simulink library "monroe_library"  (R2012b)
settings: Solver=ode45  StartTime=0.0  StopTime=10.0  RelTol=1e-3
values from neighbouring files (symbols this model uses):
  input_bit_width = ', num2str(input_bit_width))    [fft_direct_draw.m]
undefined symbols (not defined in the file or in its folder): gcbh, xlBlockLoadCallback
libraries: xbsIndex_r4 x1880, monroe_library x159, casper_library x13, xps_library x1
(part 22 of 43)

== system monroe_library/direct_coeff_gen/coeff_gen_stage_3_group_1 ==
  sync : Inport
  Concat : xbsIndex_r4/Concat  num_inputs=2  dbl_ovrd=off  block_type=concat
  Concat1 : xbsIndex_r4/Concat  num_inputs=2  dbl_ovrd=off  block_type=concat
  Concat2 : xbsIndex_r4/Concat  num_inputs=2  dbl_ovrd=off  block_type=concat
  Constant : xbsIndex_r4/Constant  arith_type=Boolean  const=0  n_bits=16  bin_pt=14  explicit_period=on  period=1  equ=P=C  opselect=C  inp2=PCIN>>17  opr=+  inp1=P  carry=CIN  dbl_ovrd=off  block_type=constant
  Constant1 : xbsIndex_r4/Constant  arith_type=Boolean  const=1  n_bits=16  bin_pt=14  explicit_period=off  period=1  equ=P=C  opselect=C  inp2=PCIN>>17  opr=+  inp1=P  carry=CIN  dbl_ovrd=off  block_type=constant
  Constant3 : xbsIndex_r4/Constant  arith_type=Signed (2's comp)  const=0  n_bits=18  bin_pt=17  explicit_period=on  period=1  equ=P=C  opselect=C  inp2=PCIN>>17  opr=+  inp1=P  carry=CIN  dbl_ovrd=off  block_type=constant
  Constant4 : xbsIndex_r4/Constant  arith_type=Boolean  const=0  n_bits=16  bin_pt=14  explicit_period=off  period=1  equ=P=C  opselect=C  inp2=PCIN>>17  opr=+  inp1=P  carry=CIN  dbl_ovrd=off  block_type=constant
  Constant5 : xbsIndex_r4/Constant  arith_type=Unsigned  const=2  n_bits=10  bin_pt=0  explicit_period=on  period=1  equ=P=C  opselect=C  inp2=PCIN>>17  opr=+  inp1=P  carry=CIN  dbl_ovrd=off  block_type=constant
  Counter : xbsIndex_r4/Counter  cnt_type=Free Running  cnt_to=Inf  operation=Up  start_count=0  cnt_by_val=1  arith_type=Unsigned  n_bits=10  bin_pt=0  load_pin=on  rst=off  en=off  explicit_period=on  period=1  dbl_ovrd=off  use_behavioral_HDL=off  implementation=Fabric  block_type=counter
  Delay : xbsIndex_r4/Delay  en=off  latency=0  dbl_ovrd=off  reg_retiming=off  block_type=delay
  Dual Port RAM4 : xbsIndex_r4/Dual Port RAM  depth=2048  initVector=[0 -0.000766990318742704 -0.00153398018628477 -0.0023009691514258 -0.00306795676296598 -0.00383494256970623 -0.00460192612044857 -0.00536890696399634 -0.00613588464915448 -0.00690285872472976 -0.0076698287395311 -0.0084367942423698 -0.00920375478205982 -0.00997070990741803 -0.0107376591672645 -0.0115046021104227 -0.0122715382857199 -0.0130384672419873 -0.0138053885280604 -0.0145723016927791 -0.0153392062849881 -0.0161061018535373 -0.0168729879472817 -0.0176398641150821 -0.0184067299058048 -0.0191735848683226 -0.0199404285515144 -0.0207072605042659 -0.0214740802754695 -0.022240887414025 -0.0230076814688394 -0.0237744619888276 -0.0245412285229123 -0.0253079806200246 -0.0260747178291039 -0.0268414396990985 -0.0276081457789657 -0.0283748356176721 -0.0291415087641937 -0.0299081647675166 -0.0306748031766366 -0.0314414235405603 -0.0322080254083046 -0.0329746083288973 -0.0337411718513776 -0.0345077155247957 -0.0352742388982139 -0.0360407415207062 -0.0368072229413588 -0.0375736827092705 -0.0383401203735527 -0.0391065354833299 -0.0398729275877398 -0.0406392962359337 -0.0414056409770767 -0.0421719613603479 -0.0429382569349408 -0.0437045272500634 -0.0444707718549387 -0.0452369902988046 -0.0460031821309146 -0.0467693469005379 -0.0475354841569593 -0.0483015934494801 -0.049067674327418 -0.0498337263401073 -0.0505997490368993 -0.0513657419671626 -0.0521317046802833 -0.0528976367256653 -0.0536635376527305 -0.0544294070109191 -0.0551952443496899 -0.0559610492185206 -0.0567268211669077 -0.0574925597443676 -0.0582582645004358 -0.0590239349846679 -0.0597895707466399 -0.0605551713359478 -0.0613207363022086 -0.0620862651950601 -0.0628517575641614 -0.0636172129591931 -0.0643826309298575 -0.0651480110258788 -0.0659133527970038 -0.0666786557930016 -0.0674439195636641 -0.0682091436588063 -0.0689743276282667 -0.0697394710219073 -0.0705045733896139 -0.0712696342812964 -0.0720346532468893 -0.0727996298363517 -0.0735645635996674 -0.0743294540868458 -0.0750943008479213 -0.0758591034329544 -0.0766238613920315 -0.077388574275265 -0.0781532416327942 -0.0789178630147849 -0.0796824379714301 -0.08044696605295 -0.0812114468095924 -0.0819758797916331 -0.0827402645493757 -0.0835046006331524 -0.0842688875933241 -0.0850331249802803 -0.0857973123444399 -0.0865614492362512 -0.0873255352061921 -0.0880895698047705 -0.0888535525825246 -0.089617483090023 -0.090381360877865 -0.091145185496681 -0.0919089564971327 -0.0926726734299133 -0.0934363358457478 -0.0941999432953932 -0.094963495329639 -0.0957269914993072 -0.0964904313552526 -0.0972538144483633 -0.0980171403295606 -0.0987804085497996 -0.0995436186600693 -0.100306770211393 -0.101069862754828 -0.101832895841467 -0.102595869022436 -0.1033587818489 -0.104121633872055 -0.104884424643135 -0.105647153713411 -0.106409820634188 -0.107172424956809 -0.107934966232654 -0.108697444013139 -0.109459857849718 -0.110222207293883 -0.110984491897163 -0.111746711211127 -0.112508864787379 -0.113270952177564 -0.114032972933367 -0.11479492660651 -0.115556812748755 -0.116318630911905 -0.117080380647801 -0.117842061508325 -0.118603673045401 -0.119365214810991 -0.120126686357102 -0.120888087235777 -0.121649416999106 -0.122410675199216 -0.12317186138828 -0.123932975118512 -0.124694015942168 -0.125454983411546 -0.12621587707899 -0.126976696496886 -0.127737441217662 -0.128498110793793 -0.129258704777796 -0.130019222722233 -0.130779664179712 -0.131540028702883 -0.132300315844445 -0.133060525157139 -0.133820656193755 -0.134580708507126 -0.135340681650134 -0.136100575175706 -0.136860388636816 -0.137620121586486 -0.138379773577784 -0.139139344163826 -0.139898832897777 -0.140658239332849 -0.141417563022303 -0.142176803519448 -0.142935960377643 -0.143695033150294 -0.14445402139086 -0.145212924652847 -0.145971742489812 -0.146730474455362 -0.147489120103154 -0.148247678986896 -0.149006150660348 -0.149764534677322 -0.150522830591677 -0.15128103795733 -0.152039156328246 -0.152797185258443 -0.153555124301993 -0.15431297301302 -0.155070730945701 ...(+33766 chars)]  distributed_mem=Block RAM  init_a=0  init_b=0  rst_a=off  rst_b=off  en_a=off  en_b=off  latency=2  write_mode_A=No Read On Write  write_mode_B=No Read On Write  dbl_ovrd=off  optimize=Area  use_rpm=on  block_type=dpram
  Reinterpret : xbsIndex_r4/Reinterpret  force_arith_type=on  arith_type=Unsigned  force_bin_pt=on  bin_pt=0  block_type=reinterpret
      settings: infoedit="Changes signal type without altering the binary representation.   You can changed the signal between signed and unsigned, and relocate the binary point.<br><br>Hardware notes: In hardware this block costs nothing.<br><br>Example:  Suppose the input is 6 bits wide, signed, with 2 fractional bits, and the output is forced to unsigned with 0 fractional bits.  Then an input of -2.0 (1110.00 in binary 2's complement) becomes an output of 56 (111000 in binary)."
  Reinterpret1 : xbsIndex_r4/Reinterpret  force_arith_type=on  arith_type=Unsigned  force_bin_pt=on  bin_pt=0  block_type=reinterpret
      settings: infoedit="Changes signal type without altering the binary representation.   You can changed the signal between signed and unsigned, and relocate the binary point.<br><br>Hardware notes: In hardware this block costs nothing.<br><br>Example:  Suppose the input is 6 bits wide, signed, with 2 fractional bits, and the output is forced to unsigned with 0 fractional bits.  Then an input of -2.0 (1110.00 in binary 2's complement) becomes an output of 56 (111000 in binary)."
  count_slice : xbsIndex_r4/Slice  nbits=10  boolean_output=off  mode=Upper Bit Location + Width  bit1=0  base1=MSB of Input  bit0=0  base0=MSB of Input  dbl_ovrd=off  block_type=slice
  coeff : Outport
  wires:
  count_slice/1 -> Concat1/2, Concat/2  "xlsub2_Counter_out1"
  Constant3/1 -> Dual Port RAM4/5, Dual Port RAM4/2  "xlsub2_Constant3_out1"
  Constant/1 -> Dual Port RAM4/6, Dual Port RAM4/3  "xlsub2_Constant_out1"
  Reinterpret1/1 -> Concat2/2  "xlsub2_Reinterpret1_out1"
  Dual Port RAM4/2 -> Reinterpret1/1  "xlsub2_Dual_Port_RAM4_out2"
  Reinterpret/1 -> Concat2/1  "xlsub2_Reinterpret_out1"
  Dual Port RAM4/1 -> Reinterpret/1  "xlsub2_Dual_Port_RAM4_out1"
  Concat1/1 -> Dual Port RAM4/4  "xlsub2_Concat1_out1"
  Concat/1 -> Dual Port RAM4/1  "xlsub2_Concat_out1"
  Delay/1 -> coeff/1
  Concat2/1 -> Delay/1  "xlsub2_Concat2_out1"
  Counter/1 -> count_slice/1
  Constant5/1 -> Counter/2  "xlsub2_Constant5_out1"
  sync/1 -> Counter/1
  Constant4/1 -> Concat1/1  "xlsub2_Constant4_out1"
  Constant1/1 -> Concat/1  "xlsub2_Constant1_out1"
